simulink library "RspLib"  (R2018b)
settings: Solver=VariableStepAuto  StartTime=0.0  StopTime=10.0  RelTol=1e-3
libraries: simulink x1
settings Model: Creator=sn2xws  LastModifiedBy=sn2xws

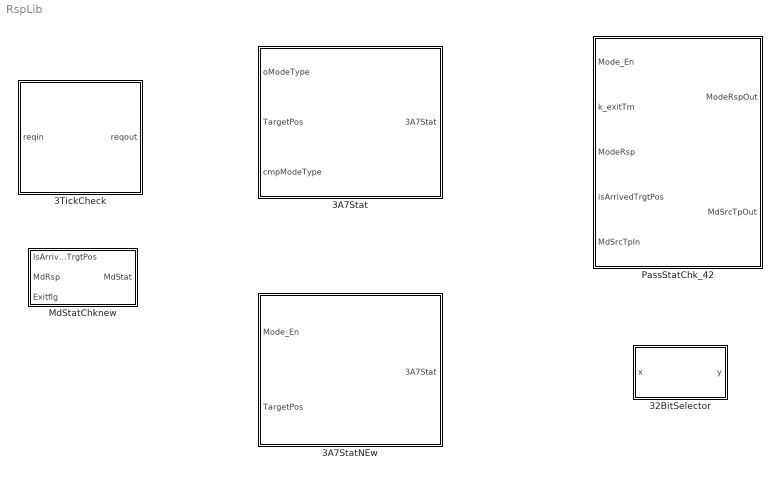
== system RspLib ==
  32BitSelector : Subsystem  mask(32 Bit Selector){BitNum=1}
      mask prompts: BitNum "Select Bit Number"
      mask help: Allows selection of a particular bit (0-31) out of a packed word up to 32 bits long. Output will be true if the bit number selected via the mask parameter is equal to one.
      mask TypeOptions BitNum: 0 | 1 | 2 | 3 | 4 | 5 | 6 | 7 | 8 | 9 | 10 | 11 | 12 | 13 | 14 | 15 | 16 | 17 | 18 | 19 | 20 | 21 | 22 | 23 | 24 | 25 | 26 | 27 | 28 | 29 | 30 | 31
      mask Display:
      | text(0.5, 0.8,'BIT','horizontalAlignment','center')
      | text(0.5, 0.5,'SELECTOR','horizontalAlignment','center')
      | text(0.5, 0.2,['-- Bit ',char(get_param(gcb,'BitNum')),' --'],'horizontalAlignment','center')
  3A7Stat : Subsystem
  3A7StatNEw : Subsystem
  3TickCheck : Subsystem
  MdStatChknew : Subsystem
  PassStatChk_42 : Stateflow chart  TreatAsAtomicUnit=on

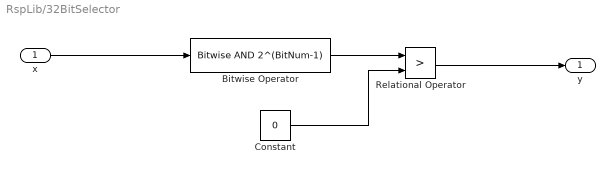
== system RspLib/32BitSelector ==
  x : Inport
  Bitwise Operator : simulink/Logic and Bit Operations/Bitwise Operator  logicop=AND  UseBitMask=on  BitMask=2^(BitNum-1)  BitMaskRealWorld=Stored Integer
  Constant : Constant  Value=0  OutDataTypeStr=uint32
  Relational Operator : RelationalOperator  Operator=>  OutDataTypeStr=boolean  RndMeth=Simplest
  y : Outport
  wires:
  Relational Operator/1 -> y/1
  Constant/1 -> Relational Operator/2
  x/1 -> Bitwise Operator/1
  Bitwise Operator/1 -> Relational Operator/1

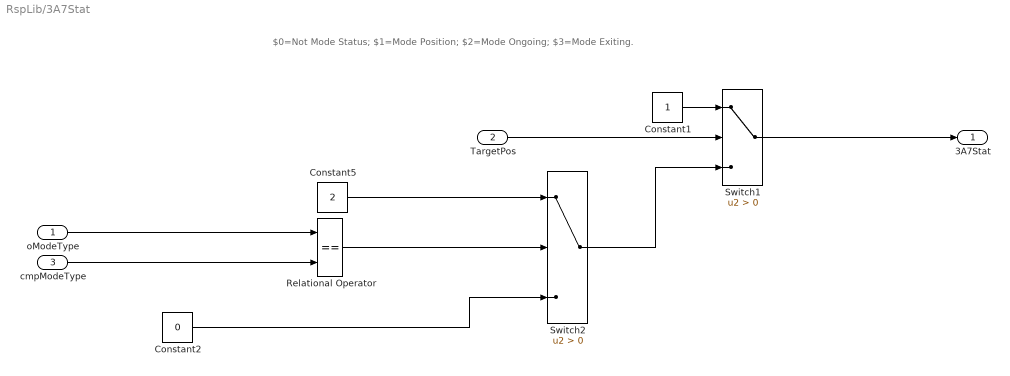
== system RspLib/3A7Stat ==
  note: $0=Not Mode Status; $1=Mode Position; $2=Mode Ongoing; $3=Mode Exiting.
  oModeType : Inport
  TargetPos : Inport  Port=2
  cmpModeType : Inport  Port=3
  Constant1 : Constant  OutDataTypeStr=uint8
  Constant2 : Constant  Value=0  OutDataTypeStr=uint8
  Constant5 : Constant  Value=2  OutDataTypeStr=uint8
  Relational Operator : RelationalOperator  Operator===  OutDataTypeStr=boolean  RndMeth=Simplest
  Switch1 : Switch  Criteria=u2 > Threshold
  Switch2 : Switch  Criteria=u2 > Threshold
  3A7Stat : Outport
  wires:
  Constant5/1 -> Switch2/1
  cmpModeType/1 -> Relational Operator/2
  TargetPos/1 -> Switch1/2
  Constant1/1 -> Switch1/1
  Relational Operator/1 -> Switch2/2
  oModeType/1 -> Relational Operator/1
  Switch1/1 -> 3A7Stat/1
  Constant2/1 -> Switch2/3
  Switch2/1 -> Switch1/3

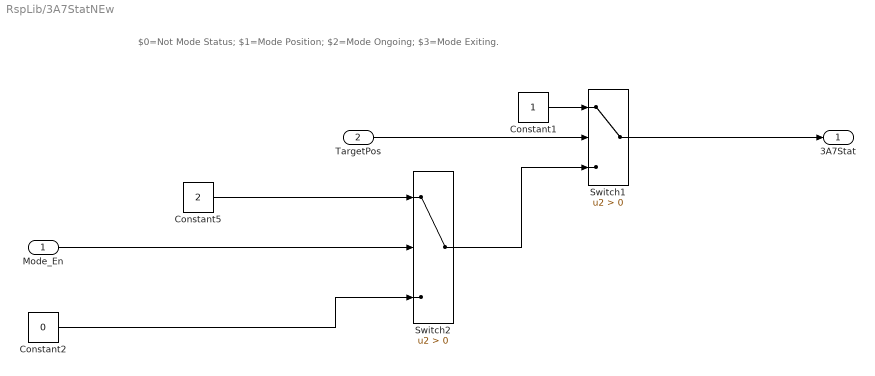
== system RspLib/3A7StatNEw ==
  note: $0=Not Mode Status; $1=Mode Position; $2=Mode Ongoing; $3=Mode Exiting.
  Mode_En : Inport
  TargetPos : Inport  Port=2
  Constant1 : Constant  OutDataTypeStr=uint8
  Constant2 : Constant  Value=0  OutDataTypeStr=uint8
  Constant5 : Constant  Value=2  OutDataTypeStr=uint8
  Switch1 : Switch  Criteria=u2 > Threshold
  Switch2 : Switch  Criteria=u2 > Threshold
  3A7Stat : Outport
  wires:
  Switch2/1 -> Switch1/3
  Constant2/1 -> Switch2/3
  Switch1/1 -> 3A7Stat/1
  Constant1/1 -> Switch1/1
  TargetPos/1 -> Switch1/2
  Constant5/1 -> Switch2/1
  Mode_En/1 -> Switch2/2

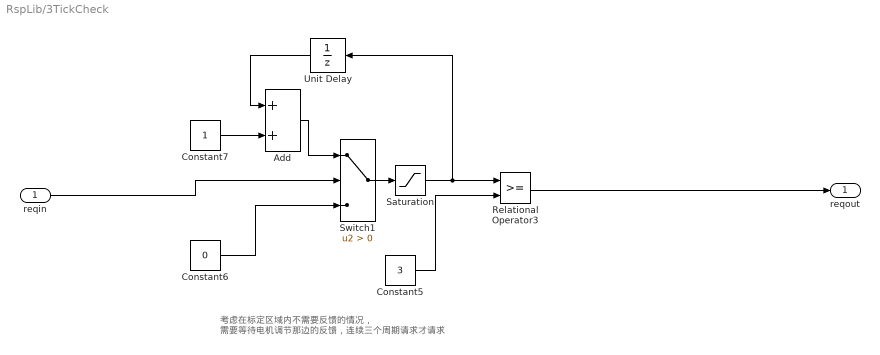
== system RspLib/3TickCheck ==
  note: 考虑在标定区域内不需要反馈的情况，
      | 需要等待电机调节那边的反馈，连续三个周期请求才请求
  reqin : Inport
  Add : Sum
  Constant5 : Constant  Value=3  OutDataTypeStr=uint8
  Constant6 : Constant  Value=0  OutDataTypeStr=uint8
  Constant7 : Constant  OutDataTypeStr=uint8
  Relational Operator3 : RelationalOperator  OutDataTypeStr=boolean  RndMeth=Simplest
  Saturation : Saturate  UpperLimit=3  LowerLimit=0  OutDataTypeStr=uint8
  Switch1 : Switch  Criteria=u2 > Threshold
  Unit Delay : UnitDelay  SampleTime=-1
  reqout : Outport
  wires:
  Unit Delay/1 -> Add/1
  Constant6/1 -> Switch1/3
  Constant5/1 -> Relational Operator3/2
  Constant7/1 -> Add/2
  Saturation/1 -> Unit Delay/1, Relational Operator3/1
  Add/1 -> Switch1/1
  Switch1/1 -> Saturation/1
  reqin/1 -> Switch1/2
  Relational Operator3/1 -> reqout/1

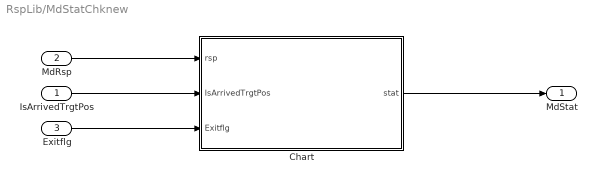
== system RspLib/MdStatChknew ==
  IsArrivedTrgtPos : Inport
  MdRsp : Inport  Port=2
  Exitflg : Inport  Port=3
  Chart : Stateflow chart  TreatAsAtomicUnit=on
  MdStat : Outport
  wires:
  MdRsp/1 -> Chart/1(rsp)
  Exitflg/1 -> Chart/3(Exitflg)
  IsArrivedTrgtPos/1 -> Chart/2(IsArrivedTrgtPos)
  Chart/1(stat) -> MdStat/1

== stateflow chart RspLib/PassStatChk_42 ==
  state othermode
    en:ModeRspOut =0;
    en:cntexit=1;
    en:MdSrcTpOut = SrcReqTp_None;
  state cmpmodeOngoing
    en:ModeRspOut =4;
    en:MdSrcTpOut = MdSrcTpIn;
  state TartPosAlready
    en:ModeRspOut =MdRsp_TargetPositionAlready;
    en:MdSrcTpOut = MdSrcTpIn;
    du:cntexit++;
  note: /*Change Request 147856
      | 在前提条件不满足、开关打断、防夹干涉导致模式中断时，
      | MSM需要先判断此模式是否已经满足调用成功的条件，
      | 若不满足，再报调用失败。210816*/
  state exitingsuccess
    en:ModeRspOut =MdRsp_RecallSuccessfully;
    du:cntexit++;
  state NotSuccessfully
    en:ModeRspOut =ModeRsp;
    du:cntexit++;
  (default) -> othermode
  othermode -> (junction 46) : [(Mode_En)]
  (junction 46) -> cmpmodeOngoing [order 2]
  (junction 46) -> TartPosAlready [order 1] : [isArrivedTrgtPos]
  TartPosAlready -> othermode : [cntexit>=k_exitTm]
  exitingsuccess -> othermode : [cntexit>=k_exitTm]
  cmpmodeOngoing -> exitingsuccess [order 1] : [(!Mode_En)&&(isArrivedTrgtPos)]
  NotSuccessfully -> othermode [order 2] : [cntexit>=k_exitTm]
  NotSuccessfully -> cmpmodeOngoing [order 1] : [Mode_En]
  cmpmodeOngoing -> NotSuccessfully [order 2] : [(!Mode_En)]
  data: Mode_En input boolean; k_exitTm input uint8; cntexit local uint8; ModeRsp input Enum: MdRspLocal2; ModeRspOut output uint8; isArrivedTrgtPos input boolean; MdSrcTpOut output Enum: SrcReqTp1; MdSrcTpIn input Enum: SrcReqTp1

== stateflow chart RspLib/MdStatChknew/Chart ==
  state idle
    en:stat = 0;
  state ongoing
    en:stat = 2;
  state ispos
    en:stat = 1;
  (default) -> idle
  idle -> ongoing [order 1] : [rsp==4]
  ongoing -> ispos [order 1] : [rsp==1]
  ongoing -> idle [order 2] : [rsp!=4]
  idle -> ispos [order 2] : [rsp==5]
  ispos -> idle : [!IsArrivedTrgtPos ||Exitflg]
  data: rsp input uint8; IsArrivedTrgtPos input boolean; Exitflg input boolean; stat output uint8
